simulink library "Library_simple_model"  (R2023b)
settings: Solver=ode45  StartTime=0.0  StopTime=10.0  RelTol=1e-3  EnableMultiTasking=on
undefined symbols (not defined in the file or in its folder): delta_param_Vert_stab_param, Flap_param_Vector
settings Model: Creator=Drago  LastModifiedBy=dragom
settings SolverCC: AlgebraicLoopSolver=TrustRegion
settings DataIOCC: LimitDataPoints=on  SaveFormat=Array  SignalLoggingSaveFormat=ModelDataLogs  ReturnWorkspaceOutputs=off
settings OptimizationCC: ExpressionDepthLimit=2147483647  LifeSpan=inf
settings DebuggingCC: UnderspecifiedInitializationDetection=Classic  MergeDetectMultiDrivingBlocksExec=none  SolverPrmCheckMsg=warning  FcnCallInpInsideContextMsg=warning  UnconnectedInputMsg=warning  UnconnectedOutputMsg=warning  UnconnectedLineMsg=warning  StateNameClashWarn=warning  SFUnexpectedBacktrackingDiag=warning  SFNoUnconditionalDefaultTransitionDiag=warning  SFExecutionAtInitializationDiag=none  ArithmeticOperatorsInVariantConditions=warning
settings HardwareCC: ProdBitPerPointer=32  ProdBitPerSizeT=32  ProdBitPerPtrDiffT=32  ProdLargestAtomicFloat=None  ProdIntDivRoundTo=Undefined  ProdEndianess=Unspecified  ProdWordSize=32  ProdHWDeviceType=32-bit Generic
settings ModelReferenceCC: PropagateSignalLabelsOutOfModel=off
settings SFSimCC: SimUseLocalCustomCode=off  CustomCodeUndefinedFunction=UseInterfaceOnly
settings RTWCC: RTWUseLocalCustomCode=off
settings CodeAppCC: StateflowObjectComments=on
settings GRTTargetCC: TargetLangStandard=C89/C90 (ANSI)  CombineOutputUpdateFcns=off  GRTInterface=on
settings ConfigComp: CovMetricSettings=dw  CovSaveCumulativeToWorkspaceVar=on  CovSaveSingleToWorkspaceVar=on  CovExternalEMLEnable=off  CovSFcnEnable=off

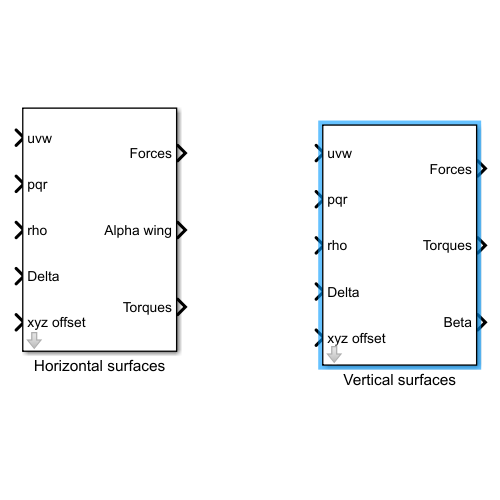
[thumbnail: Simulink's stored preview of the top-level diagram]
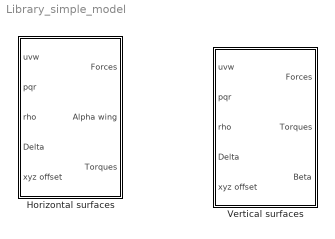
== system Library_simple_model ==
  Horizontal surfaces : Subsystem  mask{xyz_Aero=[1 1 1], S_Wing=1, Alpha_0=0, Alpha_param_Vector=[0 1 2 3], CL_param_Vector=[1 2 3 4], CD_param_Vector=[1 2 3 4]}
  Vertical surfaces : Subsystem  mask{xyzbody_Vert_stab=[1 1 1], S_Body_Vert_stab=1, beta_param_Vert_stab_param=[1 2 3 4], CY_Vert_stab_param=[1 2 3 4], CD_Vert_stab_param=[1 2 3 4]}
      mask prompts: xyzbody_Vert_stab "xyz_Vert_stab"; S_Body_Vert_stab "S_Vert_stab"; beta_param_Vert_stab_param "beta_param_Vert_stab"; CY_Vert_stab_param "CY_Vert_stab"; CD_Vert_stab_param "CD_Vert_stab"

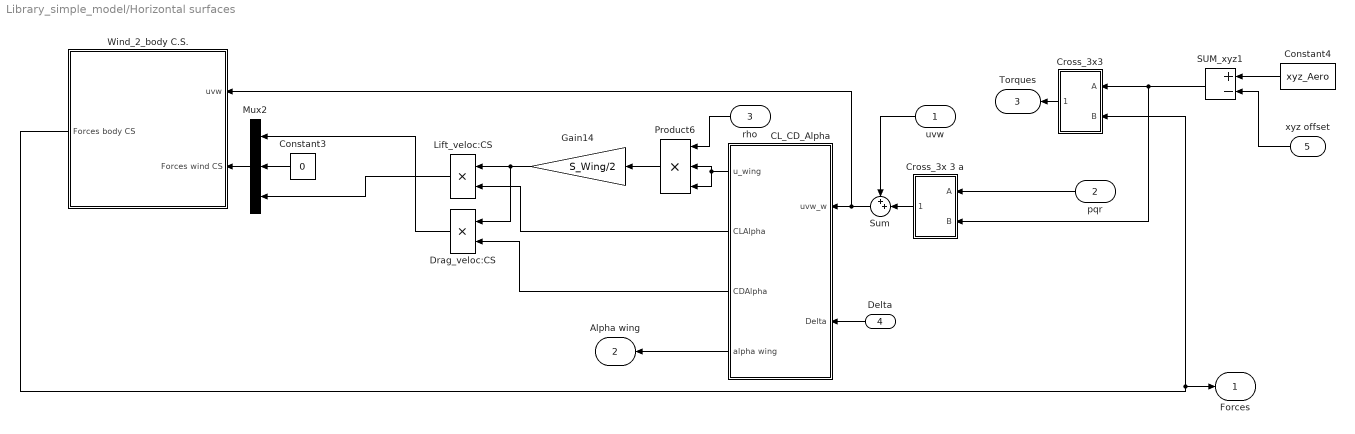
== system Library_simple_model/Horizontal surfaces ==
  uvw : Inport
  pqr : Inport  Port=2
  rho : Inport  Port=3
  Delta : Inport  Port=4
  xyz offset : Inport  Port=5
  CL_CD_Alpha : Subsystem
  Constant3 : Constant  Value=0
  Constant4 : Constant  Value=xyz_Aero
  Cross_3x 3 a : Subsystem
  Cross_3x3 : Subsystem
  Drag_veloc:CS : Product  RndMeth=Zero
  Gain14 : Gain  Gain=S_Wing/2
  Lift_veloc:CS : Product  RndMeth=Zero
  Mux2 : Mux  Inputs=3
  Product6 : Product  Inputs=3  RndMeth=Zero
  SUM_xyz1 : Sum  Inputs=+-
  Sum : Sum  Inputs=++|
  Wind_2_body C.S. : Subsystem
  Forces : Outport
  Alpha wing : Outport  Port=2
  Torques : Outport  Port=3
  wires:
  uvw/1 -> Sum/1
  pqr/1 -> Cross_3x 3 a/1(A)
  Cross_3x 3 a/1(Out1) -> Sum/2
  Delta/1 -> CL_CD_Alpha/2(Delta)
  Lift_veloc:CS/1 -> Mux2/3
  Cross_3x3/1(Torques) -> Torques/1
  Product6/1 -> Gain14/1
  CL_CD_Alpha/1(u_wing) -> Product6/2, Product6/3
  Drag_veloc:CS/1 -> Mux2/1
  CL_CD_Alpha/2(CLAlpha) -> Lift_veloc:CS/2
  rho/1 -> Product6/1
  Gain14/1 -> Lift_veloc:CS/1, Drag_veloc:CS/1
  Sum/1 -> Wind_2_body C.S./1(uvw), CL_CD_Alpha/1(uvw_w)
  CL_CD_Alpha/3(CDAlpha) -> Drag_veloc:CS/2
  Wind_2_body C.S./1("Forces body CS ") -> Cross_3x3/2(B), Forces/1
  SUM_xyz1/1 -> Cross_3x 3 a/2(B), Cross_3x3/1(A)
  Constant4/1 -> SUM_xyz1/1
  xyz offset/1 -> SUM_xyz1/2
  CL_CD_Alpha/4(alpha wing) -> Alpha wing/1
  Mux2/1 -> Wind_2_body C.S./2(Forces wind CS)
  Constant3/1 -> Mux2/2

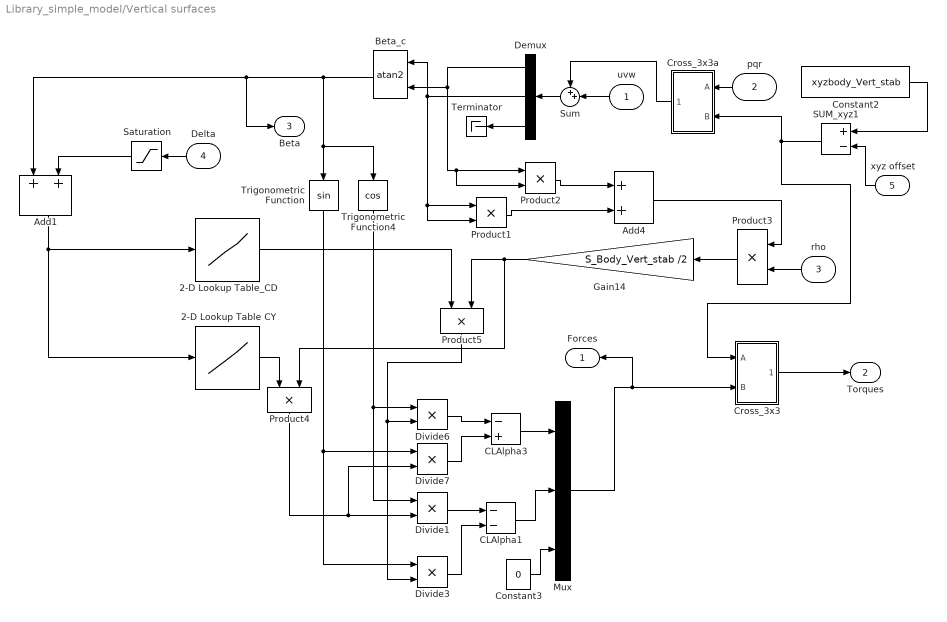
== system Library_simple_model/Vertical surfaces ==
  uvw : Inport
  pqr : Inport  Port=2
  rho : Inport  Port=3
  Delta : Inport  Port=4
  xyz offset : Inport  Port=5
  2-D Lookup Table CY : Lookup_n-D  NumberOfTableDimensions=1  BreakpointsForDimension1=beta_param_Vert_stab_param  BreakpointsForDimension2=delta_param_Vert_stab_param*pi/180  Table=CY_Vert_stab_param  InternalRulePriority=Speed  RndMeth=Simplest
  2-D Lookup Table_CD : Lookup_n-D  NumberOfTableDimensions=1  BreakpointsForDimension1=beta_param_Vert_stab_param  BreakpointsForDimension2=delta_param_Vert_stab_param*pi/180  Table=CD_Vert_stab_param  InternalRulePriority=Speed  RndMeth=Simplest
  Add1 : Sum
  Add4 : Sum
  Beta_c : Trigonometry  Operator=atan2
  CLAlpha1 : Sum  Inputs=--
  CLAlpha3 : Sum  Inputs=-+
  Constant2 : Constant  Value=xyzbody_Vert_stab
  Constant3 : Constant  Value=0
  Cross_3x3 : Subsystem
  Cross_3x3a : Subsystem
  Demux : Demux  Outputs=3
  Divide{1,3,6..7} (4 alike) : Product  Inputs=**
  Gain14 : Gain  Gain=S_Body_Vert_stab /2
  Mux : Mux  Inputs=3
  Product{1..5} (5 alike) : Product  RndMeth=Zero
  SUM_xyz1 : Sum  Inputs=+-
  Saturation : Saturate  UpperLimit=25*pi/180  LowerLimit=-25*pi/180
  Sum : Sum  Inputs=++|
  Terminator : Terminator
  Trigonometric Function : Trigonometry
  Trigonometric Function4 : Trigonometry  Operator=cos
  Forces : Outport
  Torques : Outport  Port=2
  Beta : Outport  Port=3
  wires:
  uvw/1 -> Sum/2
  Cross_3x3a/1(Out1) -> Sum/1
  SUM_xyz1/1 -> Cross_3x3a/2(B), Cross_3x3/1(A)
  pqr/1 -> Cross_3x3a/1(A)
  Sum/1 -> Demux/1
  Demux/1 -> Product2/2, Product2/1, Beta_c/2
  Demux/2 -> Beta_c/1, Product1/2, Product1/1
  Product2/1 -> Add4/1
  Add4/1 -> Product3/1
  Product1/1 -> Add4/2
  Demux/3 -> Terminator/1
  Product3/1 -> Gain14/1
  2-D Lookup Table_CD/1 -> Product5/1
  Gain14/1 -> Product4/2, Product5/2
  Product5/1 -> Divide3/2, Divide6/2
  Constant3/1 -> Mux/3
  Mux/1 -> Forces/1, Cross_3x3/2(B)
  CLAlpha1/1 -> Mux/2
  Product4/1 -> Divide1/2, Divide7/2
  Trigonometric Function4/1 -> Divide6/1, Divide1/1
  Trigonometric Function/1 -> Divide3/1, Divide7/1
  CLAlpha3/1 -> Mux/1
  Divide6/1 -> CLAlpha3/1
  Divide7/1 -> CLAlpha3/2
  Divide1/1 -> CLAlpha1/1
  Divide3/1 -> CLAlpha1/2
  rho/1 -> Product3/2
  Beta_c/1 -> Trigonometric Function/1, Trigonometric Function4/1, Add1/1, Beta/1
  2-D Lookup Table CY/1 -> Product4/1
  Delta/1 -> Saturation/1
  Cross_3x3/1(Torques) -> Torques/1
  xyz offset/1 -> SUM_xyz1/2
  Constant2/1 -> SUM_xyz1/1
  Saturation/1 -> Add1/2
  Add1/1 -> 2-D Lookup Table_CD/1, 2-D Lookup Table CY/1

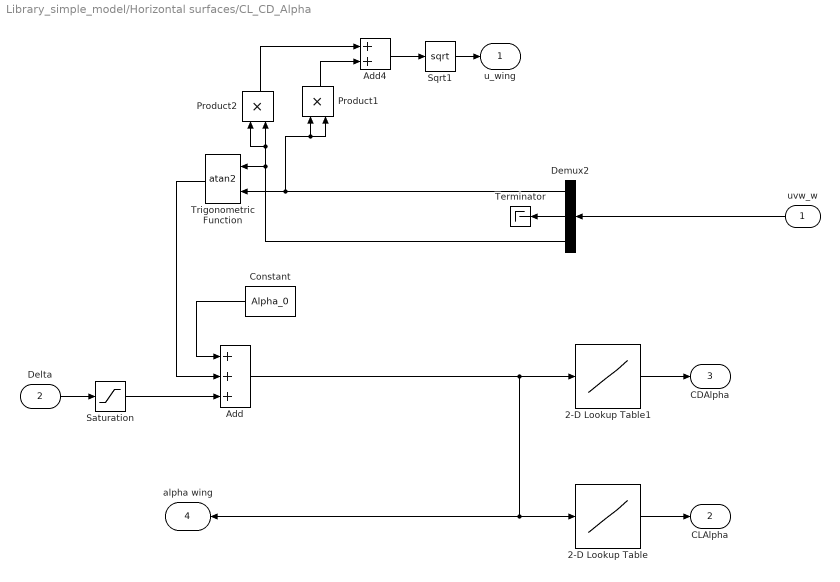
== system Library_simple_model/Horizontal surfaces/CL_CD_Alpha ==
  uvw_w : Inport
  Delta : Inport  Port=2
  2-D Lookup Table : Lookup_n-D  NumberOfTableDimensions=1  BreakpointsForDimension1=Alpha_param_Vector  BreakpointsForDimension2=Flap_param_Vector*pi/180  Table=CL_param_Vector  InternalRulePriority=Speed  RndMeth=Simplest
  2-D Lookup Table1 : Lookup_n-D  NumberOfTableDimensions=1  BreakpointsForDimension1=Alpha_param_Vector  BreakpointsForDimension2=Flap_param_Vector*pi/180  Table=CD_param_Vector  InternalRulePriority=Speed  RndMeth=Simplest
  Add : Sum  Inputs=+++
  Add4 : Sum
  Constant : Constant  Value=Alpha_0
  Demux2 : Demux  Outputs=3
  Product1 : Product  RndMeth=Zero
  Product2 : Product  RndMeth=Zero
  Saturation : Saturate  UpperLimit=25*pi/180  LowerLimit=-25*pi/180
  Sqrt1 : Sqrt
  Terminator : Terminator
  Trigonometric Function : Trigonometry  Operator=atan2
  u_wing : Outport
  CLAlpha : Outport  Port=2
  CDAlpha : Outport  Port=3
  alpha wing : Outport  Port=4
  wires:
  Demux2/3 -> Trigonometric Function/1, Product2/2, Product2/1
  Demux2/1 -> Product1/2, Product1/1, Trigonometric Function/2
  Delta/1 -> Saturation/1
  Product1/1 -> Add4/2
  Add4/1 -> Sqrt1/1
  Sqrt1/1 -> u_wing/1
  Product2/1 -> Add4/1
  Trigonometric Function/1 -> Add/2
  2-D Lookup Table1/1 -> CDAlpha/1
  2-D Lookup Table/1 -> CLAlpha/1
  Add/1 -> 2-D Lookup Table1/1, 2-D Lookup Table/1, alpha wing/1
  Constant/1 -> Add/1
  uvw_w/1 -> Demux2/1
  Demux2/2 -> Terminator/1
  Saturation/1 -> Add/3

== system Library_simple_model/Horizontal surfaces/Cross_3x 3 a ==
  A : Inport
  B : Inport  Port=2
  Subsystem : Subsystem
  Subsystem1 : Subsystem
  Sum2 : Sum  Inputs=+|-  InputSameDT=on  SaturateOnIntegerOverflow=on  OutDataTypeStr=Inherit: Same as first input
  Out1 : Outport
  wires:
  B/1 -> Subsystem/2(B1), Subsystem1/2(B1)
  Subsystem1/1(Out2) -> Sum2/2
  Subsystem/1(Out2) -> Sum2/1
  Sum2/1 -> Out1/1
  A/1 -> Subsystem1/1(A1), Subsystem/1(A1)

== system Library_simple_model/Horizontal surfaces/Cross_3x3 ==
  A : Inport
  B : Inport  Port=2
  Subsystem : Subsystem
  Subsystem1 : Subsystem
  Sum2 : Sum  Inputs=+|-  InputSameDT=on  SaturateOnIntegerOverflow=on  OutDataTypeStr=Inherit: Same as first input
  Torques : Outport
  wires:
  A/1 -> Subsystem/1(A1), Subsystem1/1(A1)
  Sum2/1 -> Torques/1
  Subsystem/1(Out2) -> Sum2/1
  Subsystem1/1(Out2) -> Sum2/2
  B/1 -> Subsystem1/2(B1), Subsystem/2(B1)

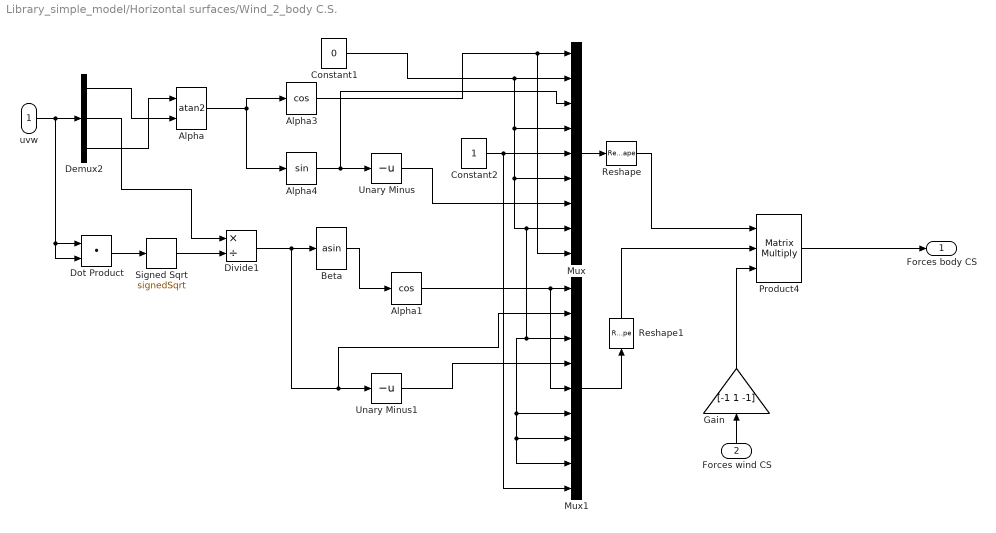
== system Library_simple_model/Horizontal surfaces/Wind_2_body C.S. ==
  uvw : Inport
  Forces wind CS : Inport  Port=2
  Alpha : Trigonometry  Operator=atan2
  Alpha1 : Trigonometry  Operator=cos
  Alpha3 : Trigonometry  Operator=cos
  Alpha4 : Trigonometry
  Beta : Trigonometry  Operator=asin
  Constant1 : Constant  Value=0
  Constant2 : Constant
  Demux2 : Demux  Outputs=3
  Divide1 : Product  Inputs=*/
  Dot Product : DotProduct  OutDataTypeStr=Inherit: Inherit via internal rule
  Gain : Gain  Gain=[-1 1 -1]
  Mux : Mux  Inputs=9
  Mux1 : Mux  Inputs=9
  Product4 : Product  Inputs=3  Multiplication=Matrix(*)
  Reshape : Reshape  OutputDimensionality=Customize  OutputDimensions=[3,3]
  Reshape1 : Reshape  OutputDimensionality=Customize  OutputDimensions=[3,3]
  Signed Sqrt : Sqrt  Operator=signedSqrt
  Unary Minus : UnaryMinus
  Unary Minus1 : UnaryMinus
  "Forces body CS " : Outport
  wires:
  Signed Sqrt/1 -> Divide1/2
  Reshape1/1 -> Product4/2
  Reshape/1 -> Product4/1
  Unary Minus1/1 -> Mux1/4
  Divide1/1 -> Mux1/2, Unary Minus1/1, Beta/1
  Alpha1/1 -> Mux1/1, Mux1/5
  Beta/1 -> Alpha1/1
  Mux1/1 -> Reshape1/1
  Dot Product/1 -> Signed Sqrt/1
  Unary Minus/1 -> Mux/7
  Constant2/1 -> Mux/5, Mux1/9
  Constant1/1 -> Mux/2, Mux/4, Mux/6, Mux/8, Mux1/8, Mux1/7, Mux1/6, Mux1/3
  Alpha3/1 -> Mux/1, Mux/9
  Alpha4/1 -> Mux/3, Unary Minus/1
  Alpha/1 -> Alpha4/1, Alpha3/1
  Mux/1 -> Reshape/1
  Demux2/1 -> Alpha/2
  Demux2/2 -> Divide1/1
  Forces wind CS/1 -> Gain/1
  uvw/1 -> Demux2/1, Dot Product/2, Dot Product/1
  Demux2/3 -> Alpha/1
  Product4/1 -> "Forces body CS "/1
  Gain/1 -> Product4/3

== system Library_simple_model/Vertical surfaces/Cross_3x3 ==
  A : Inport
  B : Inport  Port=2
  Subsystem : Subsystem
  Subsystem1 : Subsystem
  Sum2 : Sum  Inputs=+|-  InputSameDT=on  SaturateOnIntegerOverflow=on  OutDataTypeStr=Inherit: Same as first input
  Torques : Outport
  wires:
  B/1 -> Subsystem/2(B1), Subsystem1/2(B1)
  Subsystem1/1(Out2) -> Sum2/2
  Subsystem/1(Out2) -> Sum2/1
  Sum2/1 -> Torques/1
  A/1 -> Subsystem1/1(A1), Subsystem/1(A1)

== system Library_simple_model/Vertical surfaces/Cross_3x3a ==
  A : Inport
  B : Inport  Port=2
  Subsystem : Subsystem
  Subsystem1 : Subsystem
  Sum2 : Sum  Inputs=+|-  InputSameDT=on  SaturateOnIntegerOverflow=on  OutDataTypeStr=Inherit: Same as first input
  Out1 : Outport
  wires:
  B/1 -> Subsystem/2(B1), Subsystem1/2(B1)
  Subsystem1/1(Out2) -> Sum2/2
  Subsystem/1(Out2) -> Sum2/1
  Sum2/1 -> Out1/1
  A/1 -> Subsystem1/1(A1), Subsystem/1(A1)

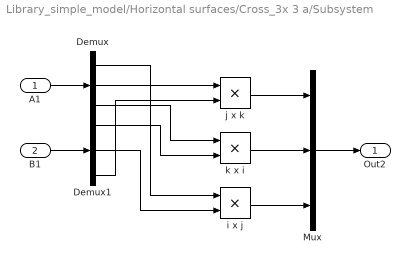
== system Library_simple_model/Horizontal surfaces/Cross_3x 3 a/Subsystem ==
  A1 : Inport
  B1 : Inport  Port=2
  Demux : Demux  Outputs=3
  Demux1 : Demux  Outputs=3
  Mux : Mux  Inputs=3
  i x j : Product  InputSameDT=on  SaturateOnIntegerOverflow=on  OutDataTypeStr=Inherit: Same as first input
  j x k : Product  InputSameDT=on  SaturateOnIntegerOverflow=on  OutDataTypeStr=Inherit: Same as first input
  k x i : Product  InputSameDT=on  SaturateOnIntegerOverflow=on  OutDataTypeStr=Inherit: Same as first input
  Out2 : Outport
  wires:
  k x i/1 -> Mux/2
  Demux1/2 -> i x j/2
  Demux1/3 -> j x k/2
  Demux1/1 -> k x i/2
  Demux/3 -> k x i/1
  Mux/1 -> Out2/1
  Demux/2 -> j x k/1
  j x k/1 -> Mux/1
  i x j/1 -> Mux/3
  B1/1 -> Demux1/1
  Demux/1 -> i x j/1
  A1/1 -> Demux/1

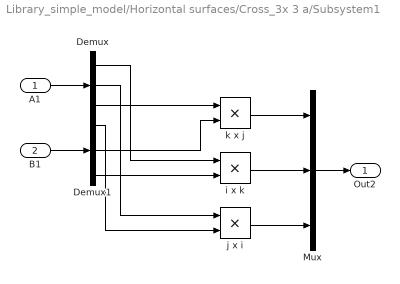
== system Library_simple_model/Horizontal surfaces/Cross_3x 3 a/Subsystem1 ==
  A1 : Inport
  B1 : Inport  Port=2
  Demux : Demux  Outputs=3
  Demux1 : Demux  Outputs=3
  Mux : Mux  Inputs=3
  i x k : Product  InputSameDT=on  SaturateOnIntegerOverflow=on  OutDataTypeStr=Inherit: Same as first input
  j x i : Product  InputSameDT=on  SaturateOnIntegerOverflow=on  OutDataTypeStr=Inherit: Same as first input
  k x j : Product  InputSameDT=on  SaturateOnIntegerOverflow=on  OutDataTypeStr=Inherit: Same as first input
  Out2 : Outport
  wires:
  j x i/1 -> Mux/3
  i x k/1 -> Mux/2
  k x j/1 -> Mux/1
  Mux/1 -> Out2/1
  Demux1/1 -> j x i/2
  Demux/2 -> j x i/1
  Demux1/3 -> i x k/2
  Demux/1 -> i x k/1
  Demux/3 -> k x j/1
  Demux1/2 -> k x j/2
  B1/1 -> Demux1/1
  A1/1 -> Demux/1

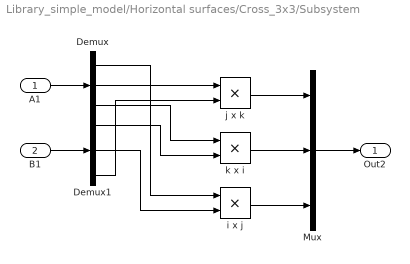
== system Library_simple_model/Horizontal surfaces/Cross_3x3/Subsystem ==
  A1 : Inport
  B1 : Inport  Port=2
  Demux : Demux  Outputs=3
  Demux1 : Demux  Outputs=3
  Mux : Mux  Inputs=3
  i x j : Product  InputSameDT=on  SaturateOnIntegerOverflow=on  OutDataTypeStr=Inherit: Same as first input
  j x k : Product  InputSameDT=on  SaturateOnIntegerOverflow=on  OutDataTypeStr=Inherit: Same as first input
  k x i : Product  InputSameDT=on  SaturateOnIntegerOverflow=on  OutDataTypeStr=Inherit: Same as first input
  Out2 : Outport
  wires:
  A1/1 -> Demux/1
  Demux/1 -> i x j/1
  B1/1 -> Demux1/1
  i x j/1 -> Mux/3
  j x k/1 -> Mux/1
  Demux/2 -> j x k/1
  Mux/1 -> Out2/1
  Demux/3 -> k x i/1
  Demux1/1 -> k x i/2
  Demux1/3 -> j x k/2
  Demux1/2 -> i x j/2
  k x i/1 -> Mux/2

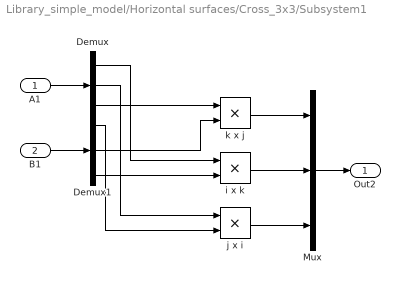
== system Library_simple_model/Horizontal surfaces/Cross_3x3/Subsystem1 ==
  A1 : Inport
  B1 : Inport  Port=2
  Demux : Demux  Outputs=3
  Demux1 : Demux  Outputs=3
  Mux : Mux  Inputs=3
  i x k : Product  InputSameDT=on  SaturateOnIntegerOverflow=on  OutDataTypeStr=Inherit: Same as first input
  j x i : Product  InputSameDT=on  SaturateOnIntegerOverflow=on  OutDataTypeStr=Inherit: Same as first input
  k x j : Product  InputSameDT=on  SaturateOnIntegerOverflow=on  OutDataTypeStr=Inherit: Same as first input
  Out2 : Outport
  wires:
  A1/1 -> Demux/1
  B1/1 -> Demux1/1
  Demux1/2 -> k x j/2
  Demux/3 -> k x j/1
  Demux/1 -> i x k/1
  Demux1/3 -> i x k/2
  Demux/2 -> j x i/1
  Demux1/1 -> j x i/2
  Mux/1 -> Out2/1
  k x j/1 -> Mux/1
  i x k/1 -> Mux/2
  j x i/1 -> Mux/3

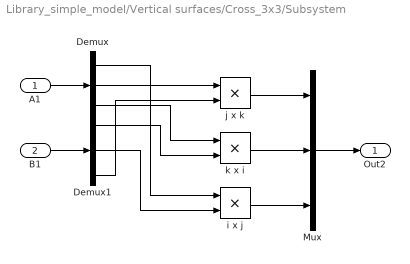
== system Library_simple_model/Vertical surfaces/Cross_3x3/Subsystem ==
  A1 : Inport
  B1 : Inport  Port=2
  Demux : Demux  Outputs=3
  Demux1 : Demux  Outputs=3
  Mux : Mux  Inputs=3
  i x j : Product  InputSameDT=on  SaturateOnIntegerOverflow=on  OutDataTypeStr=Inherit: Same as first input
  j x k : Product  InputSameDT=on  SaturateOnIntegerOverflow=on  OutDataTypeStr=Inherit: Same as first input
  k x i : Product  InputSameDT=on  SaturateOnIntegerOverflow=on  OutDataTypeStr=Inherit: Same as first input
  Out2 : Outport
  wires:
  k x i/1 -> Mux/2
  Demux1/2 -> i x j/2
  Demux1/3 -> j x k/2
  Demux1/1 -> k x i/2
  Demux/3 -> k x i/1
  Mux/1 -> Out2/1
  Demux/2 -> j x k/1
  j x k/1 -> Mux/1
  i x j/1 -> Mux/3
  B1/1 -> Demux1/1
  Demux/1 -> i x j/1
  A1/1 -> Demux/1

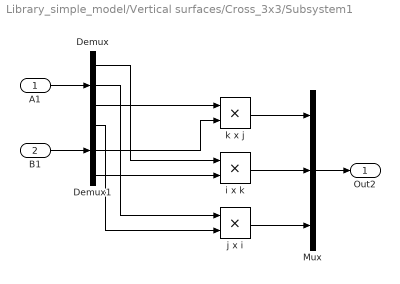
== system Library_simple_model/Vertical surfaces/Cross_3x3/Subsystem1 ==
  A1 : Inport
  B1 : Inport  Port=2
  Demux : Demux  Outputs=3
  Demux1 : Demux  Outputs=3
  Mux : Mux  Inputs=3
  i x k : Product  InputSameDT=on  SaturateOnIntegerOverflow=on  OutDataTypeStr=Inherit: Same as first input
  j x i : Product  InputSameDT=on  SaturateOnIntegerOverflow=on  OutDataTypeStr=Inherit: Same as first input
  k x j : Product  InputSameDT=on  SaturateOnIntegerOverflow=on  OutDataTypeStr=Inherit: Same as first input
  Out2 : Outport
  wires:
  j x i/1 -> Mux/3
  i x k/1 -> Mux/2
  k x j/1 -> Mux/1
  Mux/1 -> Out2/1
  Demux1/1 -> j x i/2
  Demux/2 -> j x i/1
  Demux1/3 -> i x k/2
  Demux/1 -> i x k/1
  Demux/3 -> k x j/1
  Demux1/2 -> k x j/2
  B1/1 -> Demux1/1
  A1/1 -> Demux/1

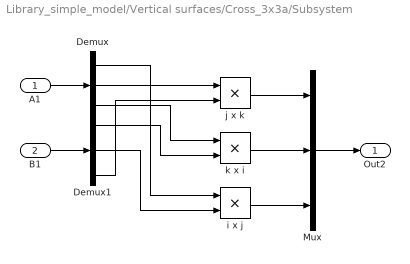
== system Library_simple_model/Vertical surfaces/Cross_3x3a/Subsystem ==
  A1 : Inport
  B1 : Inport  Port=2
  Demux : Demux  Outputs=3
  Demux1 : Demux  Outputs=3
  Mux : Mux  Inputs=3
  i x j : Product  InputSameDT=on  SaturateOnIntegerOverflow=on  OutDataTypeStr=Inherit: Same as first input
  j x k : Product  InputSameDT=on  SaturateOnIntegerOverflow=on  OutDataTypeStr=Inherit: Same as first input
  k x i : Product  InputSameDT=on  SaturateOnIntegerOverflow=on  OutDataTypeStr=Inherit: Same as first input
  Out2 : Outport
  wires:
  k x i/1 -> Mux/2
  Demux1/2 -> i x j/2
  Demux1/3 -> j x k/2
  Demux1/1 -> k x i/2
  Demux/3 -> k x i/1
  Mux/1 -> Out2/1
  Demux/2 -> j x k/1
  j x k/1 -> Mux/1
  i x j/1 -> Mux/3
  B1/1 -> Demux1/1
  Demux/1 -> i x j/1
  A1/1 -> Demux/1

== system Library_simple_model/Vertical surfaces/Cross_3x3a/Subsystem1 ==
  A1 : Inport
  B1 : Inport  Port=2
  Demux : Demux  Outputs=3
  Demux1 : Demux  Outputs=3
  Mux : Mux  Inputs=3
  i x k : Product  InputSameDT=on  SaturateOnIntegerOverflow=on  OutDataTypeStr=Inherit: Same as first input
  j x i : Product  InputSameDT=on  SaturateOnIntegerOverflow=on  OutDataTypeStr=Inherit: Same as first input
  k x j : Product  InputSameDT=on  SaturateOnIntegerOverflow=on  OutDataTypeStr=Inherit: Same as first input
  Out2 : Outport
  wires:
  j x i/1 -> Mux/3
  i x k/1 -> Mux/2
  k x j/1 -> Mux/1
  Mux/1 -> Out2/1
  Demux1/1 -> j x i/2
  Demux/2 -> j x i/1
  Demux1/3 -> i x k/2
  Demux/1 -> i x k/1
  Demux/3 -> k x j/1
  Demux1/2 -> k x j/2
  B1/1 -> Demux1/1
  A1/1 -> Demux/1
